simulink model "BufferTest"  (R2024b)
settings: Solver=ode4  StartTime=0.0  StopTime=100  FixedStep=0.001  RelTol=1e-3
undefined symbols (not defined in the file or in its folder): alpha, beta
libraries: dspstat3 x2, cstblocks x1
settings Model: Creator=kadir  LastModifiedBy=kadir

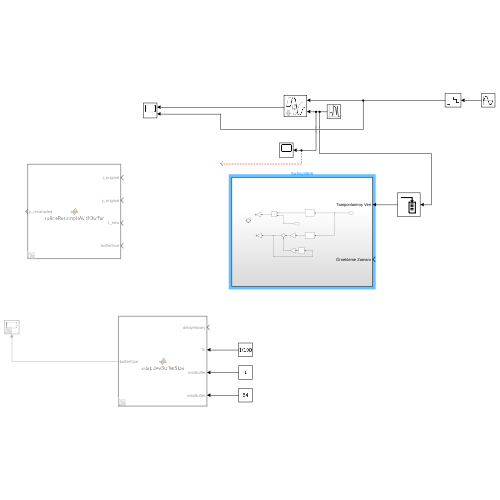
[thumbnail: Simulink's stored preview of the top-level diagram]
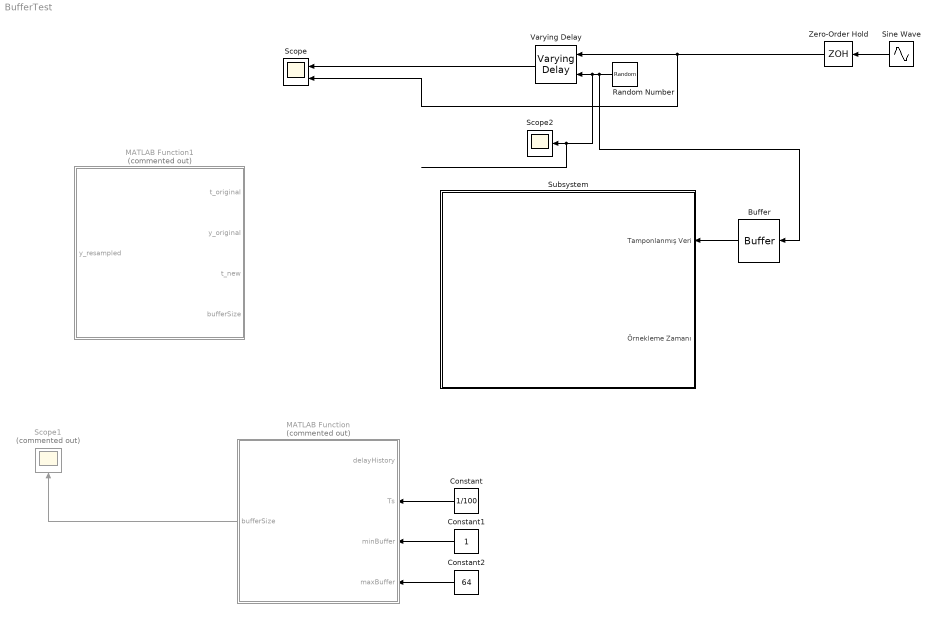
== system BufferTest ==
  Buffer : Buffer  N=128  OutputFrames=off
  Constant : Constant  Value=1/100
  Constant1 : Constant
  Constant2 : Constant  Value=64
  MATLAB Function : MATLAB Function  Commented=on  TreatAsAtomicUnit=on
  MATLAB Function1 : MATLAB Function  Commented=on  TreatAsAtomicUnit=on
  Random Number : RandomNumber  Mean=0.002  Variance=0.0001  SampleTime=0.01
  Scope : Scope  NumInputPorts=2
  Scope1 : Scope  Commented=on
  Scope2 : Scope
  Sine Wave : Sin  SampleTime=0
  Subsystem : Subsystem
  Varying Delay : cstblocks/Linear Parameter Varying/Varying Delay  Td=0  TdMax=10  TdMin=0  TdFixed=[]  u0=0  bufsize=1024  FixedBuffer=off  PadeOrder=0
  Zero-Order Hold : ZeroOrderHold  SampleTime=0.01
  wires:
  Constant2/1 -> MATLAB Function/4(maxBuffer)
  Constant/1 -> MATLAB Function/2(Ts)
  Random Number/1 -> Buffer/1, Scope2/1, Varying Delay/2
  Constant1/1 -> MATLAB Function/3(minBuffer)
  MATLAB Function/1(bufferSize) -> Scope1/1
  Sine Wave/1 -> Zero-Order Hold/1
  Varying Delay/1 -> Scope/1
  Zero-Order Hold/1 -> Varying Delay/1, Scope/2
  Buffer/1 -> Subsystem/1(Tamponlanmış Veri)

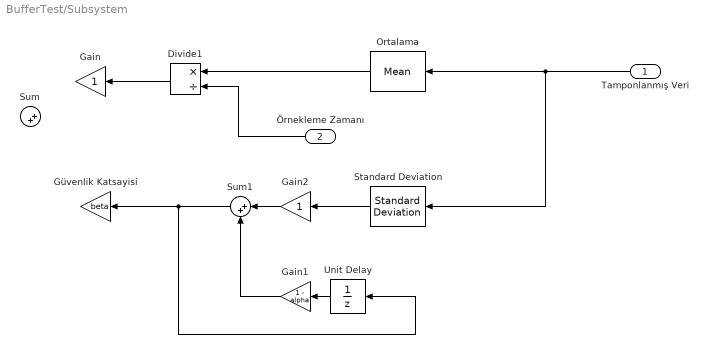
== system BufferTest/Subsystem ==
  Tamponlanmış Veri : Inport
  Örnekleme Zamanı : Inport  Port=2
  Divide1 : Product  Inputs=*/
  Gain : Gain
  Gain1 : Gain  Gain=1 - alpha
  Gain2 : Gain
  Güvenlik Katsayisi : Gain  Gain=beta
  Ortalama : dspstat3/Mean  run=off  InputProcessing=Columns as channels (frame based)  reset_popup=None  directionMode=Entire input  dimension=1  roiEnable=off  roiType=Rectangles  roiPortion=Entire ROI  roiOutput=Individual statistics for each ROI  roiFlag=off  roundingMode=Floor  overflowMode=off  outputDataTypeStr=Inherit: Same as accumulator  outputMin=[]  outputMax=[]  outputLastDataTypeStr=Inherit: Same as accumulator
  Standard Deviation : dspstat3/Standard Deviation  run=off  directionMode=Each column  dimension=1  InputProcessing=Columns as channels (frame based)  reset_popup=None  roiEnable=off  roiType=Rectangles  roiPortion=Entire ROI  roiOutput=Individual statistics for each ROI  roiFlag=off
  Sum : Sum  Inputs=|++
  Sum1 : Sum  Inputs=|++
  Unit Delay : UnitDelay  SampleTime=-1  HasFrameUpgradeWarning=on
  wires:
  Ortalama/1 -> Divide1/1
  Tamponlanmış Veri/1 -> Standard Deviation/1, Ortalama/1
  Standard Deviation/1 -> Gain2/1
  Örnekleme Zamanı/1 -> Divide1/2
  Divide1/1 -> Gain/1
  Unit Delay/1 -> Gain1/1
  Gain2/1 -> Sum1/1
  Gain1/1 -> Sum1/2
  Sum1/1 -> Güvenlik Katsayisi/1, Unit Delay/1

== matlab function BufferTest/MATLAB Function1 ==
  data: t_original input; y_resampled output; y_original input; t_new input; bufferSize input
function y_resampled = splineResampleWithBuffer(t_original, y_original, t_new, bufferSize)
%#codegen
% Resample signal using cubic spline interpolation with adaptive buffer size
% t_original: vector [Nx1] - tüm zaman geçmişi
% y_original: vector [Nx1] - tüm sinyal geçmişi
% t_new: vector [Mx1] - yeniden örnekleme zamanları
% bufferSize: int - kullanılacak veri sayısı (son bufferSize kadar)

% Ensure column vectors
t_original = t_original(:);
y_original = y_original(:);
t_new = t_new(:);

% Verinin boyutunu kontrol et (güvenlik için)
N = length(t_original);
if bufferSize > N
    bufferSize = N;
end

% Sadece son bufferSize kadar veriyi al
t_used = t_original(end-bufferSize+1:end);
y_used = y_original(end-bufferSize+1:end);

% Spline interpolasyonu uygula
y_resampled = spline(t_used, y_used, t_new);

end

== matlab function BufferTest/MATLAB Function ==
  data: delayHistory input; bufferSize output; Ts input; minBuffer input; maxBuffer input
function bufferSize = adaptiveBufferSize(delayHistory, Ts, minBuffer, maxBuffer)
    % Adaptive buffer size calculation for NCS
    % delayHistory: Gecikme ölçümlerinin vektörü (seconds)
    % Ts: Örnekleme Zamanı (saniye)
    % minBuffer, maxBuffer: Tampon bölgenin boyutu (paket sayısı)
    
    % Parametreler
    k1 = 0.8;   % Ortalama Gecikmenin Ağırlığı
    k2 = 1.2;   % Jitter Etkisinin Ağırlığı
    
    % Gecikme hesapları
    meanDelay = mean(delayHistory);
    stdDelay  = std(delayHistory);
    
    % Base buffer (at least 2 samples)
    baseSize = 2;
    
    % Yeni tampon boyutu hesaplama
    bufferSize = baseSize + k1 * (meanDelay / Ts) + k2 * (stdDelay / Ts);
    
    % Yuvarlama
    bufferSize = round(bufferSize);
    
    % Apply limits
    bufferSize = max(minBuffer, min(bufferSize, maxBuffer));
end
